simulink model "reference_model_for_fit_attitude"  (R2017b)
settings: Solver=FixedStepAuto  StartTime=0.0  StopTime=40  FixedStep=0.5  RelTol=1e-3
InitFcn:
  | % RM.angles0 = deg2rad([30, 30, -30]);
  | % RM.q0 = flip(angle2quat(RM.angles0(1),RM.angles0(2),RM.angles0(3))); %MRPs
  | % RM.s0 = RM.q0(1:3)/(1+RM.q0(4)); %verify MRP
  | % % %convert to quats using
  | % % %[t1 t2 t3] = quat2angle(flip(mrp2quat(RM.s0')'))
  | %
  | %
  | % RM.w0 = deg2rad([ 6, -6, 6])';
  | % s = RM.s0';
  | % s_tilde = [0, -s(3), s(2); s(3), 0, -s(1); -s(2), s(1), 0];
  | % SRotL = eye(3) + (8*s_tilde^2  - 4*(1-s'*s)* s_tilde )/(1 + s'*s)^2;
  | % C = (1 - s'*s)*eye(3) + 2*s_tilde + 2*(s*s');
  | % params.Rorbit = 9800;
  | % params.mu = 398600;
  | % n = sqrt(params.mu/params.Rorbit^3); % angular velocity of the LRF
  | % wL = [0;0;n];
  | % RM.s0_dot = 0.25*C*(RM.w0 - SRotL * wL);
  | 
  | % K3 = diag([0.1, 0.06, 0.096]);
  | % K4 = e-3*diag([3.7, 1.3, 3.7]);
  | % [t1, t2, t3] = quat2angle(flip(mrp2quat(Xs_out.Data'))')
  | % t1 = t1*180/pi;
  | % t2 = t2*180/pi;
  | % t3 = t3*180/pi;
settings Model: Creator=Reza  LastModifiedBy=Reza
settings OptimizationCC: DefaultParameterBehavior=Inlined  UseDivisionForNetSlopeComputation=on  UseFloatMulNetSlope=on  InlineInvariantSignals=on  PassReuseOutputArgsAs=Individual arguments  ZeroExternalMemoryAtStartup=off  ZeroInternalMemoryAtStartup=off  NoFixptDivByZeroProtection=on  EfficientFloat2IntCast=on  LifeSpan=1
settings DebuggingCC: ParameterTunabilityLossMsg=error
settings HardwareCC: ProdLongLongMode=on
settings SFSimCC: MATLABDynamicMemAlloc=off
settings RTWCC: SystemTargetFile=ert.tlc  TemplateMakefile=ert_default_tmf  GenerateReport=on  IncludeHyperlinkInReport=on  LaunchReport=on  TargetLang=C++  GenerateTraceInfo=on  GenerateTraceReport=on  GenerateTraceReportSl=on  GenerateTraceReportSf=on  GenerateTraceReportEml=on
settings CodeAppCC: ForceParamTrailComments=on  IgnoreCustomStorageClasses=off  OperatorAnnotations=on  SimulinkDataObjDesc=on  SFDataObjDesc=on  CustomSymbolStrGlobalVar=rt$N$M  CustomSymbolStrType=$N$M  CustomSymbolStrFcn=$N$M$F  CustomSymbolStrMacro=$N$M  InsertBlockDesc=on
settings ERTTargetCC: TargetLangStandard=C++03 (ISO)  GenerateSampleERTMain=on  IncludeMdlTerminateFcn=off  CombineSignalStateStructs=on  SupportAbsoluteTime=off  MultiInstanceERTCode=on  CodeInterfacePackaging=C++ class  SupportComplex=off  SupportContinuousTime=on  InlinedParameterPlacement=NonHierarchical  RootIOFormat=Structure reference  ERTCustomFileTemplate=example_file_process.tlc  ERTFilePackagingFormat=CompactWithDataFile

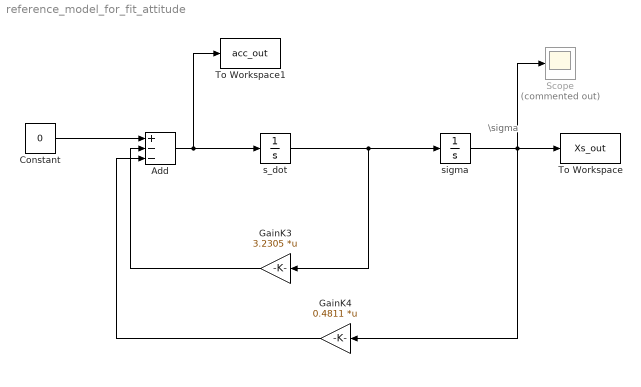
== system reference_model_for_fit_attitude ==
  note: \sigma
  Add : Sum  Inputs=+--
  Constant : Constant  Value=0
  GainK3 : Gain  Gain=3.2305  Multiplication=Matrix(K*u)
  GainK4 : Gain  Gain=0.4811  Multiplication=Matrix(K*u)
  Scope : Scope  Commented=on
  To Workspace : ToWorkspace  VariableName=Xs_out  SaveFormat=Timeseries  SampleTime=-1
  To Workspace1 : ToWorkspace  VariableName=acc_out  SaveFormat=Timeseries  SampleTime=-1
  s_dot : Integrator
  sigma : Integrator  InitialCondition=-0.16253
  wires:
  Constant/1 -> Add/1
  GainK3/1 -> Add/2
  s_dot/1 -> GainK3/1, sigma/1
  Add/1 -> To Workspace1/1, s_dot/1
  GainK4/1 -> Add/3
  sigma/1 -> Scope/1, To Workspace/1, GainK4/1
